simulink model "RealModelControlWithChopper"  (R2021a)
settings: Solver=VariableStepAuto  StartTime=0.0  StopTime=1  RelTol=1e-3
libraries: spsDCVoltageSourceLib x2, spsIGBTDiodeLib x2, spsDCMachineLib x1, pid_lib x1, spspowerguiLib x1
settings Model: Creator=User  LastModifiedBy=User

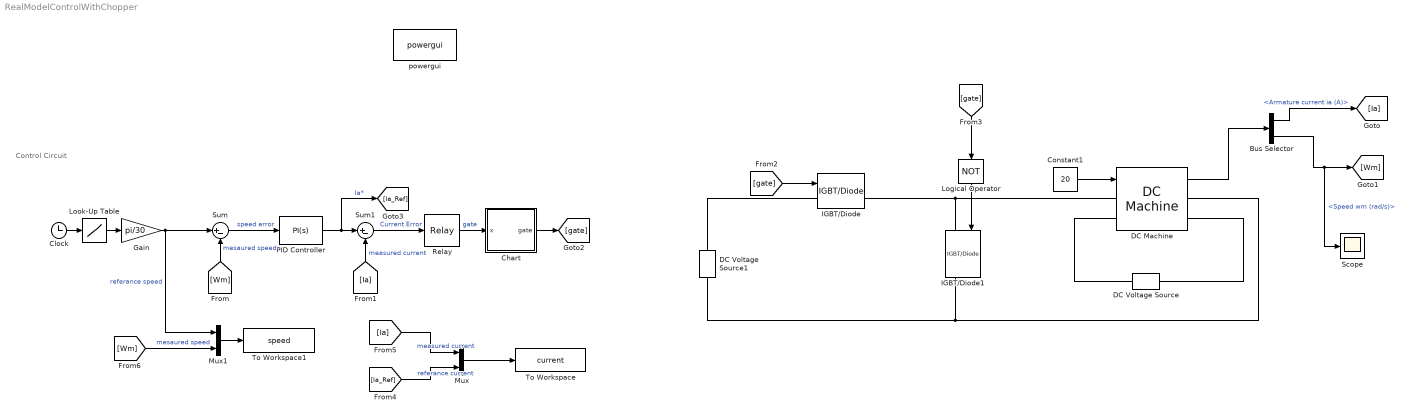
== system RealModelControlWithChopper ==
  note: Control Circuit
  Bus Selector : BusSelector  OutputSignals=Armature current ia (A),Speed wm (rad/s)
  Chart : Stateflow chart  TreatAsAtomicUnit=on
  Clock : Clock
  Constant1 : Constant  Value=20
  DC Machine : spsDCMachineLib/DC Machine  PresetModel=01: 5HP 240V 1750RPM Field:300V  MechanicalLoad=Torque TL  FieldType=Wound  ShowDetailedParameters=on  MeasurementBus=off  RLa=[2.581 0.028]  RLf=[281.2 156]  Laf=0.9483  MachineConstant=Torque constant (N.m/A)  Ke=1.8  Kt=1.8  J=0.02215  Bm=0.002953  Tf=0.5161  w0=1  Ifinit=1.06685633001422  TsPowergui=0  TsBlock=-1
  DC Voltage Source : spsDCVoltageSourceLib/DC Voltage Source  Amplitude=300  Measurements=None
  DC Voltage Source1 : spsDCVoltageSourceLib/DC Voltage Source  Amplitude=300  Measurements=None
  Gain : Gain  Gain=pi/30
  IGBT/Diode : spsIGBTDiodeLib/IGBT//Diode  Ron=1e-3  Rs=1e5  Cs=inf  Measurements=on
  IGBT/Diode1 : spsIGBTDiodeLib/IGBT//Diode  Ron=1e-3  Rs=1e5  Cs=inf  Measurements=on
  Logical Operator : Logic  Operator=NOT  AllPortsSameDT=off  OutDataTypeStr=boolean
  Look-Up Table : Lookup  InputValues=[0 .03 .03 .08 0.1 0.5 0.6 0.8]  Table=[1000 1000 1000 1500 1500 1750 1750 1750]  SaturateOnIntegerOverflow=on
  Mux : Mux  Inputs=2
  Mux1 : Mux  Inputs=2
  PID Controller : pid_lib/PID Controller  Controller=PI  Form=Parallel  TimeDomain=Continuous-time  UseExternalTs=off  SampleTime=-1  IntegratorMethod=Forward Euler  FilterMethod=Forward Euler  ControllerParametersSource=internal  P=1.5  I=100  D=0  UseFilter=on  N=100  TunerSelectOption=Transfer Function Based (PID Tuner App)  InitialConditionSource=internal  InitialConditionForIntegrator=0  InitialConditionForFilter=0  DifferentiatorICPrevScaledInput=0  ExternalReset=none  TrackingMode=off  Kt=1  LimitOutput=off  SatLimitsSource=internal  UpperSaturationLimit=15.5  LowerSaturationLimit=0  LinearizeAsGain=on  AntiWindupMode=none  Kb=1  POutMin=[]  POutMax=[]  IOutMin=[]  IOutMax=[]  DOutMin=[]  DOutMax=[]  NOutMin=[]  NOutMax=[]  SumOutMin=[]  SumOutMax=[]  SaturationOutMin=[]  SaturationOutMax=[]  PParamMin=[]  PParamMax=[]  IParamMin=[]  IParamMax=[]  DParamMin=[]  DParamMax=[]  NParamMin=[]  NParamMax=[]  KbParamMin=[]  KbParamMax=[]  KtParamMin=[]  KtParamMax=[]  KbOutMin=[]  KbOutMax=[]  KtOutMin=[]  KtOutMax=[]  IntegratorOutMin=[]  IntegratorOutMax=[]  FilterOutMin=[]  FilterOutMax=[]  SumI1OutMin=[]  SumI1OutMax=[]  SumI2OutMin=[]  SumI2OutMax=[]  SumI3OutMin=[]  SumI3OutMax=[]  SumI4OutMin=[]  SumI4OutMax=[]  SumDOutMin=[]  SumDOutMax=[]  DifferentiatorOutMin=[]  DifferentiatorOutMax=[]  FilterDiffOutCoefMin=[]  FilterDiffOutCoefMax=[]  ReciprocalOutMin=[]  ReciprocalOutMax=[]  SumDenOutMin=[]  SumDenOutMax=[]  SumNumOutMin=[]  SumNumOutMax=[]  DivideOutMin=[]  DivideOutMax=[]  UdiffTsProdOutMin=[]  UdiffTsProdOutMax=[]  NTsProdOutMin=[]  NTsProdOutMax=[]  UintegralTsProdOutMin=[]  UintegralTsProdOutMax=[]  UngainTsProdOutMin=[]  UngainTsProdOutMax=[]  IntegratorContinuousStateAttributes=''  IntegratorStateMustResolveToSignalObject=off  IntegratorRTWStateStorageClass=Auto  FilterContinuousStateAttributes=''  FilterStateMustResolveToSignalObject=off  FilterRTWStateStorageClass=Auto  ParallelPVariant=InternalParameters  IdealPVariant=Disabled  IVariant=InternalParameters  DVariant=Disabled  IntegratorVariant=Continuous  SatVariant=Disabled  AWVariant=Passthrough  PCopyVariant=Disabled  TRVariant=Disabled  FdbkBlocksVariant=Forward  IdealPFdbkVariant=Disabled  SatFdbkVariant=Disabled  DerivativeFilterVariant=Disabled  NVariant=Disabled  NCopyVariant=Disabled_SignalSpec  FilterICVariant=Disabled  IntegratorICVariant=InternalICs  ExternalResetVariant=Disabled  TRSumVariant=Passthrough  SumFdbkVariant=Disabled  SumVariant=Sum_PI  TsampFilterVariant=InternalTs  TsampNgainVariant=Passthrough  TsampIntegralVariant=Passthrough  ExternalSaturationOutDataTypeStr=Inherit: Same as second input
  Relay : Relay  OnSwitchValue=2  OffSwitchValue=-2  OnOutputValue=240
  Scope : Scope
  Sum : Sum  Inputs=|+-
  Sum1 : Sum  Inputs=|+-
  To Workspace : ToWorkspace  VariableName=current  SaveFormat=Timeseries  SampleTime=-1
  To Workspace1 : ToWorkspace  VariableName=speed  SaveFormat=Timeseries  SampleTime=-1
  powergui : spspowerguiLib/powergui  Priority=1  SimulationMode=Continuous  SampleTime=50e-6  frequency=60  Iterations=50  frequencyindice=0  Pbase=100e6  ErrMax=1e-4  UnitsV=kV  UnitsW=MW  buscounter=0  FunctionMessages=off  echomessages=off  EnableUseOfTLC=off  CurrentSourceSwitches=off  DisableSnubberDevices=off  DisableRonSwitches=off  DisableVfSwitches=off  DisplayEquations=off  AutomaticDiscreteSolvers=off  SolverType=Tustin/Backward Euler (TBE)  Interpol=off  ExternalGateDelay=off  methode=off  Ts=100  x0status=blocks  SPID=on  SwTol=0  HookPort=off  NonlinearTolerance=1e-4  nMaxIteration=100  ContinueOnMaxIteration=off  RestoreLinks=warning  ResistiveCurrentMeasurement=off  Frange=[0:2:500]  Ylog=off  Xlog=on  ShowGrid=off  save=off  variable=ZData  structure=0  ZoomFFT=off  StartTime=0.0  cycles=1  DisplayStyle=1  fundamental=60  FreqAxis=off  MaxFrequency=1000  frequencyindicesteady=1  RmsSteady=1  display=off
  wires:
  Constant1/1 -> DC Machine/1
  Clock/1 -> Look-Up Table/1
  Relay/1 -> Chart/1(x)  "gate"
  [Ia] -> Sum1/2  "measured current"
  [Wm] -> Sum/2  "mesaured speed"
  Sum/1 -> PID Controller/1  "speed error"
  PID Controller/1 -> [Ia_Ref], Sum1/1  "Ia*"
  Sum1/1 -> Relay/1  "Current Error"
  [gate] -> IGBT/Diode/1
  DC Machine/1 -> Bus Selector/1
  Bus Selector/1 -> [Ia]  "<Armature current ia (A)>"
  Bus Selector/2 -> Scope/1, [Wm]  "<Speed wm (rad/s)>"
  Gain/1 -> Sum/1, Mux1/1  "referance speed"
  Look-Up Table/1 -> Gain/1
  [gate] -> Logical Operator/1
  Logical Operator/1 -> IGBT/Diode1/1
  Chart/1(gate) -> [gate]
  [Ia_Ref] -> Mux/2  "referance current"
  Mux/1 -> To Workspace/1
  Mux1/1 -> To Workspace1/1
  [Ia] -> Mux/1  "measured current"
  [Wm] -> Mux1/2  "mesaured speed"
  connections:
  DC Machine/RConn1 -- DC Voltage Source1/LConn1 -- IGBT/Diode1/RConn1
  IGBT/Diode/RConn1 -- IGBT/Diode1/LConn1 -- DC Machine/LConn1
  DC Voltage Source/RConn1 -- DC Machine/LConn2
  DC Voltage Source1/RConn1 -- IGBT/Diode/LConn1
  DC Voltage Source/LConn1 -- DC Machine/RConn2

== stateflow chart RealModelControlWithChopper/Chart ==
  (default) -> (junction 7) : % switching
  (junction 7) -> (junction 8) [order 1] : [x == 240]
  (junction 7) -> (junction 9) [order 2] : {gate=0;}
  (junction 8) -> (junction 10) : {gate =1;}
  (junction 10) -> (junction 9)
  (junction 9) -> (junction 11)
  data: x input; gate output
